simulink model "DCM_UnitTest"  (R2018b)
settings: Solver=VariableStepAuto  StartTime=0.0  StopTime=10.0  RelTol=1e-3
libraries: Rotations x3
settings Model: Creator=IvanMachuca  LastModifiedBy=IvanMachuca

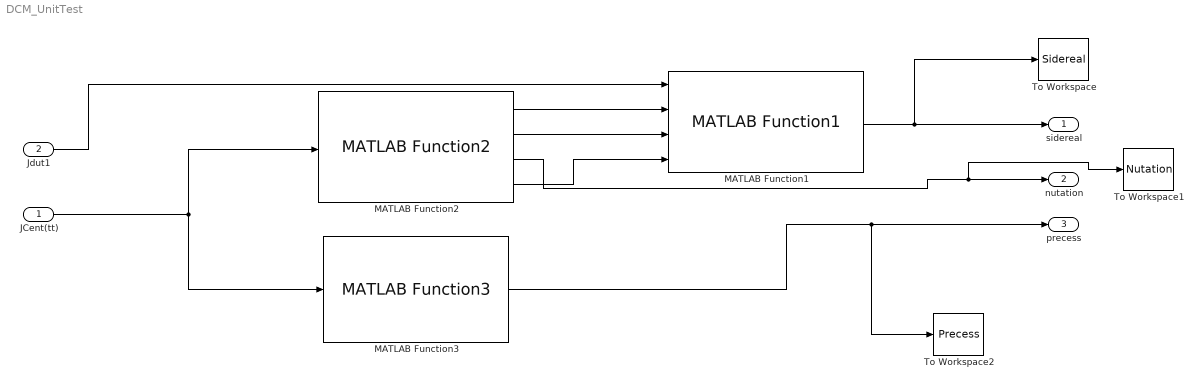
== system DCM_UnitTest ==
  "JCent(tt) " : Inport
  Jdut1 : Inport  Port=2
  MATLAB Function1 : Rotations/MATLAB Function1  SystemSampleTime=-1
  MATLAB Function2 : Rotations/MATLAB Function2  SystemSampleTime=-1
  MATLAB Function3 : Rotations/MATLAB Function3  SystemSampleTime=-1
  To Workspace : ToWorkspace  VariableName=Sidereal  SampleTime=-1
      settings: Save2DSignal=2-D array (concatenate along first dimension)
  To Workspace1 : ToWorkspace  VariableName=Nutation  SampleTime=-1
  To Workspace2 : ToWorkspace  VariableName=Precess  SampleTime=-1
      settings: Save2DSignal=2-D array (concatenate along first dimension)
  "sidereal " : Outport
  "nutation " : Outport  Port=2
  "precess " : Outport  Port=3
  wires:
  MATLAB Function2/1 -> MATLAB Function1/2
  MATLAB Function2/2 -> MATLAB Function1/3
  Jdut1/1 -> MATLAB Function1/1
  "JCent(tt) "/1 -> MATLAB Function3/1, MATLAB Function2/1
  MATLAB Function2/4 -> MATLAB Function1/4
  MATLAB Function1/1 -> To Workspace/1, "sidereal "/1
  MATLAB Function2/3 -> To Workspace1/1, "nutation "/1
  MATLAB Function3/1 -> To Workspace2/1, "precess "/1
